simulink model "B2_SIM"  (R2024a)
settings: Solver=VariableStepAuto  StartTime=0.0  StopTime=1200  RelTol=1e-3
values from neighbouring files (symbols this model uses):
  alpha1 = 0.03198    [diseased_prm.m]
  alpha2 = 0.05591    [diseased_prm.m]
  beta1 = 0.008275    [diseased_prm.m]
  beta2 = 0.03255    [diseased_prm.m]
  CaCO2_IC = 0.565    [diseased_prm.m]
  CaO2_IC = 0.184    [diseased_prm.m]
  CsatCO2 = 1.9488    [diseased_prm.m]
  CsatO2 = 0.2128    [diseased_prm.m]
  CvCO2_IC = 0.602    [diseased_prm.m]
  CvO2_IC = 0.134    [diseased_prm.m]
  h1 = 0.3836    [diseased_prm.m]
  h2 = 1.819    [diseased_prm.m]
  K = 11.5620    (= 11.562)    [B2.m]
  K1 = 15.0    (= 15)    [diseased_prm.m]
  K2 = 194.4    [diseased_prm.m]
  kEff = 0.55    [diseased_prm.m]
  kem = 0.192    [diseased_prm.m]
  MRCO2 = 3.30/1000    (= 0.0033)    [diseased_prm.m]
  MRO2 = 3.80/1000    (= 0.0038)    [diseased_prm.m]
  PACO2_IC = 55.0    (= 55)    [diseased_prm.m]
  PAO2_IC = 57.0    (= 57)    [diseased_prm.m]
  Patm = 760.0    (= 760)    [diseased_prm.m]
  PdCO2_IC = 53.0    (= 53)    [diseased_prm.m]
  PdO2_IC = 60.0    (= 60)    [diseased_prm.m]
  PECO2_IC = 40.0    (= 40)    [diseased_prm.m]
  PEO2_IC = 200.0    (= 200)    [diseased_prm.m]
  PICO2 = (Patm - Pws)*FICO2    (= 0)    [diseased_prm.m]
  PIO2 = (Patm - Pws)*FIO2    (= 713)    [diseased_prm.m]
  Pws = 47.0    (= 47)    [diseased_prm.m]
  R = 10.0    (= 10)    [diseased_prm.m]
  Rlung = 1.4013    [diseased_prm.m]
  Rtube = 3.76    [diseased_prm.m]
  shunt = 36.5/100    (= 0.365)    [diseased_prm.m]
  Tau_LT = 18.0    (= 18)    [diseased_prm.m]
  Tau_TL = 10.0    (= 10)    [diseased_prm.m]
  Tsamp = 1e-3    (= 0.001)    [diseased_prm.m]
  VD = 0.15    [diseased_prm.m]
  VECO2 = 1.5    [diseased_prm.m]
  VEO2 = 1.5    [diseased_prm.m]
  VprimeEcmo = 0.08    [B2.m]
  VReference = 0.2    [B2.m]    (also in diseased_prm.m = 0.6)
  VTCO2 = 6000/1000    (= 6)    [diseased_prm.m]
  VTO2 = 7700/1000    (= 7.7)    [diseased_prm.m]
libraries: fl_lib x14, nesl_utility x7, slpidlib x4, ee_lib x2
settings Model: Creator=seman  LastModifiedBy=seman

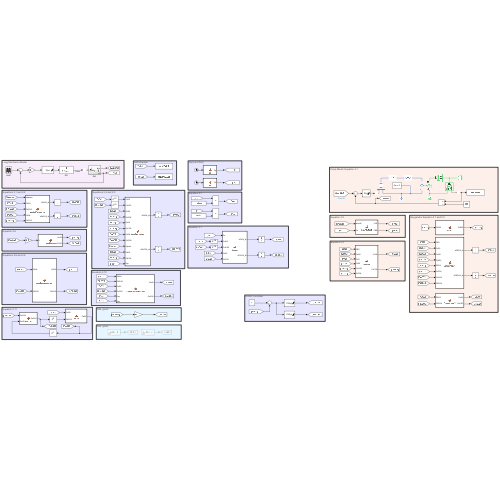
[thumbnail: Simulink's stored preview of the top-level diagram]
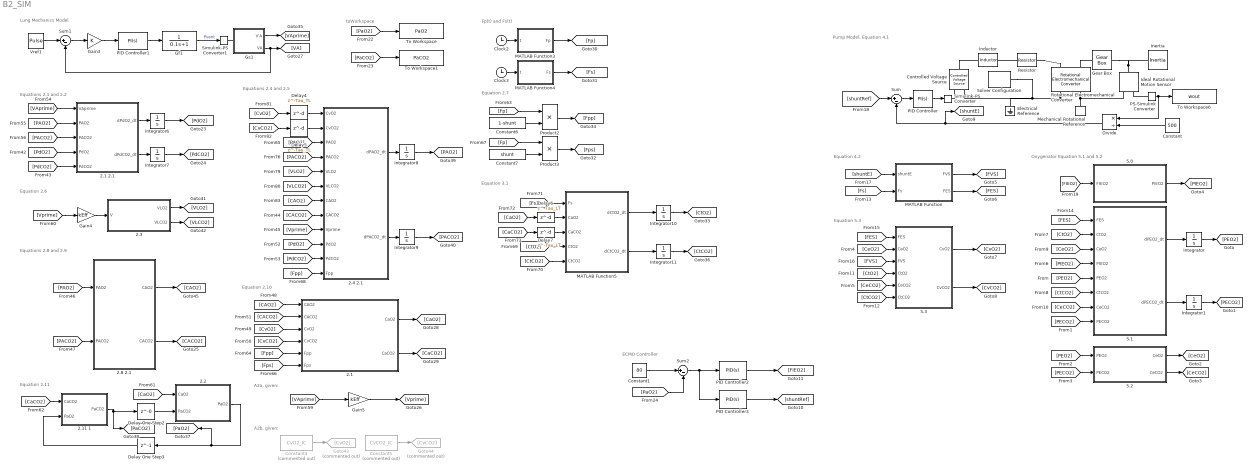
== system B2_SIM ==
  note: ECMO Controller
  note: Equation 5.3
  note: Oxygenator Equation 5.1 and 5.2
  note: Equation 4.2
  note: Equation 2.7
  note: Lung Mechanics Model
  note: Equation 2.6
  note: Equations 2.8 and 2.9
  note: A2b, given:
  note: Equation 2.11
  note: toWorkspace
  note: Fp(t) and Fs(t)
  note: Equations 2.1 and 2.2
  note: Equations 2.4 and 2.5
  note: Equation 3.1
  note: Equation 2.10
  note: A2a, given:
  note: Pump Model, Equation 4.1
  " 2.11 1" : MATLAB Function  TreatAsAtomicUnit=on  SystemSampleTime=Tsamp
  2.1 : MATLAB Function  TreatAsAtomicUnit=on  SystemSampleTime=Tsamp
  2.1 2.1 : MATLAB Function  TreatAsAtomicUnit=on  SystemSampleTime=Tsamp
  2.2 : MATLAB Function  TreatAsAtomicUnit=on  SystemSampleTime=Tsamp
  2.3 : MATLAB Function  TreatAsAtomicUnit=on  SystemSampleTime=Tsamp
  2.4 2.1 : MATLAB Function  TreatAsAtomicUnit=on  SystemSampleTime=Tsamp
  2.8 2.1 : MATLAB Function  TreatAsAtomicUnit=on  SystemSampleTime=Tsamp
  5.0 : MATLAB Function  TreatAsAtomicUnit=on  SystemSampleTime=Tsamp
  5.1 : MATLAB Function  TreatAsAtomicUnit=on  SystemSampleTime=Tsamp
  5.2 : MATLAB Function  TreatAsAtomicUnit=on  SystemSampleTime=Tsamp
  5.3 : MATLAB Function  TreatAsAtomicUnit=on  SystemSampleTime=Tsamp
  Clock2 : Clock
  Clock3 : Clock
  Constant : Constant  Value=500
  Constant1 : Constant  Value=80
  Constant4 : Constant  Commented=on  Value=CvO2_IC  SampleTime=Tsamp
  Constant5 : Constant  Commented=on  Value=CvCO2_IC  SampleTime=Tsamp
  Constant6 : Constant  Value=1-shunt
  Constant7 : Constant  Value=shunt
  Controlled Voltage Source : fl_lib/Electrical/Electrical Sources/Controlled Voltage Source
  Delay One Step2 : Delay  DelayLength=0  InitialCondition=PACO2_IC  SampleTime=Tsamp
  Delay One Step3 : Delay  DelayLength=1  InitialCondition=PAO2_IC  SampleTime=Tsamp
  Delay4 : Delay  DelayLength=Tau_TL  InitialCondition=CvO2_IC  SampleTime=Tsamp
  Delay5 : Delay  DelayLength=Tau_TL  InitialCondition=CvCO2_IC  SampleTime=Tsamp
  Delay6 : Delay  DelayLength=Tau_LT  InitialCondition=CaO2_IC  SampleTime=Tsamp
  Delay7 : Delay  DelayLength=Tau_LT  InitialCondition=CaCO2_IC  SampleTime=Tsamp
  Divide : Product  Inputs=*/
  Electrical Reference : fl_lib/Electrical/Electrical Elements/Electrical Reference
  Gain3 : Gain  Gain=K
  Gain4 : Gain  Gain=kEff
  Gain5 : Gain  Gain=kEff
  Gear Box : fl_lib/Mechanical/Mechanisms/Gear Box  ratio=Ng  t_in_specify=off  t_in_priority=None  t_in=0 N*m  t_in_nominal_specify=off  t_in_nominal_value=1  t_in_nominal_unit=N*m  t_out_specify=off  t_out_priority=None  t_out=0 N*m  t_out_nominal_specify=off  t_out_nominal_value=1  t_out_nominal_unit=N*m
  Gf1 : TransferFcn  Denominator=[0.1 1]
  Goto43 : Goto  Commented=on  GotoTag=CvO2
  Goto44 : Goto  Commented=on  GotoTag=CvCO2
  Gs1 : Subsystem
      settings: PortSchema="{\"entries\":[{\"content\":{\"sides\":[{\"content\":{\"connectorIds\":[\"Out1\",\"Out2\"]},\"type\":\"ConnectorPlacement.EquallySpacedRectSide\",\"uuid\":\"c27d9928-4b86-4da3-a78c-9004074cc1dc\"},{\"content\":{\"connectorIds\":[\"RConn1\"],\"side\":\"RIGHT\"},\"type\":\"ConnectorPlacement.EquallySpacedRectSide\",\"uuid\":\"e53dfbe0-a76d-428f-9787-aeb453f7ae86\"},{\"content\":{\"side\":\"TOP\"},\"type\":\"ConnectorPlacement.EquallySpacedRectSide\",\"uuid\":\"62f67270-c149-475e-8334-fb9ed6626660\"}]},\"type\":\"ConnectorPlacement.EquallySpacedConnector\",\"uuid\":\"79b18274-f0e6-497d-aef4-92df5a9879dd\"}],\"packageUris\":[\"http://schema.mathworks.com/mf0/Connector/R2020b\"],\"version\":\"1.0\"}"
  Ideal Rotational Motion Sensor : fl_lib/Mechanical/Mechanical Sensors/Ideal Rotational Motion Sensor  reference=foundation.enum.MeasurementReference.difference  acceleration_port=false  velocity_port=true  position_port=false  wrap_angle=false  offset=0 rad
      settings: InternalSimscapePortConfiguration="{\"Bottom\":[],\"Left\":[{\"id\":\"R\",\"label\":\"R\",\"type\":\"foundation.mechanical.rotational.rotational\"}],\"Right\":[{\"id\":\"C\",\"label\":\"C\",\"type\":\"foundation.mechanical.rotational.rotational\"},{\"id\":\"W\",\"label\":\"W\",\"type\":\"output\"}],\"Top\":[]}"
  Inductor : ee_lib/Passive/Inductor  l=L mH  enable_L_tol=ee.enum.toleranceApplication.none  L_tol=20  tol_distribution=ee.enum.toleranceDistribution.uniform  nSigma=4  r=0 Ohm  g=1e-9 1/Ohm  enable_operating_limits=ee.enum.enable.no  operating_limit_action=ee.enum.passive.reportOpLim.warn  max_working_current=1 A  power_rating=1 W  enable_faults=ee.enum.enable.no  fault_action=simscape.enum.assert.action.none  lambdaPercent=50  k_faulted=0.9999  turnsShort=ee.enum.passive.inductor.turnsShortOption.no  openCct=ee.enum.enable.no  groundShort=ee.enum.passive.inductor.groundShortOption.no  groundShortG=0 1/Ohm  tau_fault=1e-3 s  fault_trigger=ee.enum.faults.faultTrigger.temporal  t_fault=1 s  max_permissible_voltage=100 V  n_fail_on_voltage=1  max_permissible_current=1 A  t_fail_on_current=1 s  i_L_specify=off  i_L_priority=High  i_L=0 A  i_L_nominal_specify=off  i_L_nominal_value=1  i_L_nominal_unit=A  faulted_specify=off  faulted_priority=None  faulted=0
  Inertia : fl_lib/Mechanical/Rotational Elements/Inertia  inertia=JL kg*m^2  num_ports=foundation.enum.numPorts2.one  w_specify=off  w_priority=High  w=0 rad/s  w_nominal_specify=off  w_nominal_value=1  w_nominal_unit=rad/s  t_specify=off  t_priority=None  t=0 N*m  t_nominal_specify=off  t_nominal_value=1  t_nominal_unit=N*m
  Integrator : Integrator  InitialCondition=PEO2_IC
  Integrator1 : Integrator  InitialCondition=PECO2_IC
  Integrator10 : Integrator  InitialCondition=CvO2_IC
  Integrator11 : Integrator  InitialCondition=CvCO2_IC
  Integrator6 : Integrator  InitialCondition=PdO2_IC
  Integrator7 : Integrator  InitialCondition=PdCO2_IC
  Integrator8 : Integrator  InitialCondition=PAO2_IC
  Integrator9 : Integrator  InitialCondition=PACO2_IC
  MATLAB Function : MATLAB Function  TreatAsAtomicUnit=on  SystemSampleTime=Tsamp
  MATLAB Function3 : MATLAB Function  TreatAsAtomicUnit=on  SystemSampleTime=Tsamp
  MATLAB Function4 : MATLAB Function  TreatAsAtomicUnit=on  SystemSampleTime=Tsamp
  MATLAB Function5 : MATLAB Function  TreatAsAtomicUnit=on  SystemSampleTime=Tsamp
  Mechanical Rotational Reference : fl_lib/Mechanical/Rotational Elements/Mechanical Rotational Reference
  PID Controller : slpidlib/PID Controller  Controller=PI  Form=Parallel  TimeDomain=Continuous-time  UseExternalTs=off  SampleTime=-1  IntegratorMethod=Forward Euler  FilterMethod=Forward Euler  ControllerParametersSource=internal  P=24.7  I=48.35  UseKiTs=off  D=0  UseExternalDerivativeSource=off  N=100  UseFilter=on  TunerSelectOption=Transfer Function Based (PID Tuner App)  InitialConditionSource=internal  InitialConditionForIntegrator=0  InitialConditionForFilter=0  DifferentiatorICPrevScaledInput=0  ExternalReset=none  TrackingMode=off  Kt=1  LimitOutput=on  SatLimitsSource=internal  UpperSaturationLimit=48  LowerSaturationLimit=0  LinearizeAsGain=on  AntiWindupMode=none  Kb=1  LimitIntegrator=off  UpperIntegratorSaturationLimit=inf  LowerIntegratorSaturationLimit=-inf  POutMin=[]  POutMax=[]  IOutMin=[]  IOutMax=[]  DOutMin=[]  DOutMax=[]  NOutMin=[]  NOutMax=[]  SumOutMin=[]  SumOutMax=[]  SaturationOutMin=[]  SaturationOutMax=[]  PParamMin=[]  PParamMax=[]  IParamMin=[]  IParamMax=[]  DParamMin=[]  DParamMax=[]  NParamMin=[]  NParamMax=[]  KbParamMin=[]  KbParamMax=[]  KtParamMin=[]  KtParamMax=[]  KbOutMin=[]  KbOutMax=[]  KtOutMin=[]  KtOutMax=[]  IntegratorOutMin=[]  IntegratorOutMax=[]  FilterOutMin=[]  FilterOutMax=[]  SumI1OutMin=[]  SumI1OutMax=[]  SumI2OutMin=[]  SumI2OutMax=[]  SumI3OutMin=[]  SumI3OutMax=[]  SumI4OutMin=[]  SumI4OutMax=[]  SumDOutMin=[]  SumDOutMax=[]  DifferentiatorOutMin=[]  DifferentiatorOutMax=[]  FilterDiffOutCoefMin=[]  FilterDiffOutCoefMax=[]  ReciprocalOutMin=[]  ReciprocalOutMax=[]  SumDenOutMin=[]  SumDenOutMax=[]  SumNumOutMin=[]  SumNumOutMax=[]  DivideOutMin=[]  DivideOutMax=[]  UdiffTsProdOutMin=[]  UdiffTsProdOutMax=[]  NTsProdOutMin=[]  NTsProdOutMax=[]  UintegralTsProdOutMin=[]  UintegralTsProdOutMax=[]  UngainTsProdOutMin=[]  UngainTsProdOutMax=[]  ClampingZeroOutDataTypeStr=Inherit: Inherit via back propagation  ClampingZeroOutMin=[]  ClampingZeroOutMax=[]  FilterDenConstantOutDataTypeStr=Inherit: Inherit via back propagation  FilterDenConstantOutMin=[]  FilterDenConstantOutMax=[]  PCopyOutDataTypeStr=Inherit: Inherit via back propagation  PCopyOutMin=[]  PCopyOutMax=[]  NCopyOutDataTypeStr=Inherit: Inherit via back propagation  NCopyOutMin=[]  NCopyOutMax=[]  IntegratorContinuousStateAttributes=''  IntegratorStateMustResolveToSignalObject=off  IntegratorRTWStateStorageClass=Auto  FilterContinuousStateAttributes=''  FilterStateMustResolveToSignalObject=off  FilterRTWStateStorageClass=Auto  ParallelPVariant=InternalParameters  IdealPVariant=Disabled  IVariant=InternalParameters  DVariant=Disabled  IntegratorVariant=Continuous  SatVariant=Enabled  AWVariant=Passthrough  PCopyVariant=Disabled  TRVariant=Disabled  FdbkBlocksVariant=Forward  IdealPFdbkVariant=Disabled  SatFdbkVariant=Disabled  DerivativeFilterVariant=Disabled  NVariant=Disabled  NCopyVariant=Disabled_SignalSpec  FilterICVariant=Disabled  IntegratorICVariant=InternalICs  ExternalResetVariant=Disabled  TRSumVariant=Passthrough  SumFdbkVariant=Disabled  SumVariant=Sum_PI  TsampFilterVariant=InternalTs  TsampNgainVariant=Passthrough  TsampIntegralVariant=Disabled_SignalSpec  ExternalSaturationOutDataTypeStr=Inherit: Same as second input  DerivativeSourceVariant=Disabled
  PID Controller1 : slpidlib/PID Controller  Controller=PI  Form=Parallel  TimeDomain=Continuous-time  UseExternalTs=off  SampleTime=-1  IntegratorMethod=Forward Euler  FilterMethod=Forward Euler  ControllerParametersSource=internal  P=1  I=3.125  UseKiTs=off  D=0  UseExternalDerivativeSource=off  N=100  UseFilter=on  TunerSelectOption=Transfer Function Based (PID Tuner App)  InitialConditionSource=internal  InitialConditionForIntegrator=0  InitialConditionForFilter=0  DifferentiatorICPrevScaledInput=0  ExternalReset=none  TrackingMode=off  Kt=1  LimitOutput=on  SatLimitsSource=internal  UpperSaturationLimit=inf  LowerSaturationLimit=0  LinearizeAsGain=on  AntiWindupMode=back-calculation  Kb=1  LimitIntegrator=off  UpperIntegratorSaturationLimit=inf  LowerIntegratorSaturationLimit=-inf  POutMin=[]  POutMax=[]  IOutMin=[]  IOutMax=[]  DOutMin=[]  DOutMax=[]  NOutMin=[]  NOutMax=[]  SumOutMin=[]  SumOutMax=[]  SaturationOutMin=[]  SaturationOutMax=[]  PParamMin=[]  PParamMax=[]  IParamMin=[]  IParamMax=[]  DParamMin=[]  DParamMax=[]  NParamMin=[]  NParamMax=[]  KbParamMin=[]  KbParamMax=[]  KtParamMin=[]  KtParamMax=[]  KbOutMin=[]  KbOutMax=[]  KtOutMin=[]  KtOutMax=[]  IntegratorOutMin=[]  IntegratorOutMax=[]  FilterOutMin=[]  FilterOutMax=[]  SumI1OutMin=[]  SumI1OutMax=[]  SumI2OutMin=[]  SumI2OutMax=[]  SumI3OutMin=[]  SumI3OutMax=[]  SumI4OutMin=[]  SumI4OutMax=[]  SumDOutMin=[]  SumDOutMax=[]  DifferentiatorOutMin=[]  DifferentiatorOutMax=[]  FilterDiffOutCoefMin=[]  FilterDiffOutCoefMax=[]  ReciprocalOutMin=[]  ReciprocalOutMax=[]  SumDenOutMin=[]  SumDenOutMax=[]  SumNumOutMin=[]  SumNumOutMax=[]  DivideOutMin=[]  DivideOutMax=[]  UdiffTsProdOutMin=[]  UdiffTsProdOutMax=[]  NTsProdOutMin=[]  NTsProdOutMax=[]  UintegralTsProdOutMin=[]  UintegralTsProdOutMax=[]  UngainTsProdOutMin=[]  UngainTsProdOutMax=[]  ClampingZeroOutDataTypeStr=Inherit: Inherit via back propagation  ClampingZeroOutMin=[]  ClampingZeroOutMax=[]  FilterDenConstantOutDataTypeStr=Inherit: Inherit via back propagation  FilterDenConstantOutMin=[]  FilterDenConstantOutMax=[]  PCopyOutDataTypeStr=Inherit: Inherit via back propagation  PCopyOutMin=[]  PCopyOutMax=[]  NCopyOutDataTypeStr=Inherit: Inherit via back propagation  NCopyOutMin=[]  NCopyOutMax=[]  IntegratorContinuousStateAttributes=''  IntegratorStateMustResolveToSignalObject=off  IntegratorRTWStateStorageClass=Auto  FilterContinuousStateAttributes=''  FilterStateMustResolveToSignalObject=off  FilterRTWStateStorageClass=Auto  ParallelPVariant=InternalParameters  IdealPVariant=Disabled  IVariant=InternalParameters  DVariant=Disabled  IntegratorVariant=Continuous  SatVariant=Enabled  AWVariant=BackCalculation  PCopyVariant=Disabled  TRVariant=Disabled  FdbkBlocksVariant=Forward  IdealPFdbkVariant=Disabled  SatFdbkVariant=Disabled  DerivativeFilterVariant=Disabled  NVariant=Disabled  NCopyVariant=Disabled_SignalSpec  FilterICVariant=Disabled  IntegratorICVariant=InternalICs  ExternalResetVariant=Disabled  TRSumVariant=Passthrough  SumFdbkVariant=Disabled  SumVariant=Sum_PI  TsampFilterVariant=InternalTs  TsampNgainVariant=Passthrough  TsampIntegralVariant=Disabled_SignalSpec  ExternalSaturationOutDataTypeStr=Inherit: Same as second input  DerivativeSourceVariant=Disabled
  PID Controller2 : slpidlib/PID Controller  Controller=PID  Form=Parallel  TimeDomain=Continuous-time  UseExternalTs=off  SampleTime=-1  IntegratorMethod=Forward Euler  FilterMethod=Forward Euler  ControllerParametersSource=internal  P=1  I=0.1  UseKiTs=off  D=0.2  UseExternalDerivativeSource=off  N=100  UseFilter=on  TunerSelectOption=Transfer Function Based (PID Tuner App)  InitialConditionSource=internal  InitialConditionForIntegrator=0.2  InitialConditionForFilter=0.2  DifferentiatorICPrevScaledInput=0  ExternalReset=none  TrackingMode=off  Kt=1  LimitOutput=on  SatLimitsSource=internal  UpperSaturationLimit=1  LowerSaturationLimit=0.2  LinearizeAsGain=on  AntiWindupMode=none  Kb=1  LimitIntegrator=off  UpperIntegratorSaturationLimit=inf  LowerIntegratorSaturationLimit=-inf  POutMin=[]  POutMax=[]  IOutMin=[]  IOutMax=[]  DOutMin=[]  DOutMax=[]  NOutMin=[]  NOutMax=[]  SumOutMin=[]  SumOutMax=[]  SaturationOutMin=[]  SaturationOutMax=[]  PParamMin=[]  PParamMax=[]  IParamMin=[]  IParamMax=[]  DParamMin=[]  DParamMax=[]  NParamMin=[]  NParamMax=[]  KbParamMin=[]  KbParamMax=[]  KtParamMin=[]  KtParamMax=[]  KbOutMin=[]  KbOutMax=[]  KtOutMin=[]  KtOutMax=[]  IntegratorOutMin=[]  IntegratorOutMax=[]  FilterOutMin=[]  FilterOutMax=[]  SumI1OutMin=[]  SumI1OutMax=[]  SumI2OutMin=[]  SumI2OutMax=[]  SumI3OutMin=[]  SumI3OutMax=[]  SumI4OutMin=[]  SumI4OutMax=[]  SumDOutMin=[]  SumDOutMax=[]  DifferentiatorOutMin=[]  DifferentiatorOutMax=[]  FilterDiffOutCoefMin=[]  FilterDiffOutCoefMax=[]  ReciprocalOutMin=[]  ReciprocalOutMax=[]  SumDenOutMin=[]  SumDenOutMax=[]  SumNumOutMin=[]  SumNumOutMax=[]  DivideOutMin=[]  DivideOutMax=[]  UdiffTsProdOutMin=[]  UdiffTsProdOutMax=[]  NTsProdOutMin=[]  NTsProdOutMax=[]  UintegralTsProdOutMin=[]  UintegralTsProdOutMax=[]  UngainTsProdOutMin=[]  UngainTsProdOutMax=[]  ClampingZeroOutDataTypeStr=Inherit: Inherit via back propagation  ClampingZeroOutMin=[]  ClampingZeroOutMax=[]  FilterDenConstantOutDataTypeStr=Inherit: Inherit via back propagation  FilterDenConstantOutMin=[]  FilterDenConstantOutMax=[]  PCopyOutDataTypeStr=Inherit: Inherit via back propagation  PCopyOutMin=[]  PCopyOutMax=[]  NCopyOutDataTypeStr=Inherit: Inherit via back propagation  NCopyOutMin=[]  NCopyOutMax=[]  IntegratorContinuousStateAttributes=''  IntegratorStateMustResolveToSignalObject=off  IntegratorRTWStateStorageClass=Auto  FilterContinuousStateAttributes=''  FilterStateMustResolveToSignalObject=off  FilterRTWStateStorageClass=Auto  ParallelPVariant=InternalParameters  IdealPVariant=Disabled  IVariant=InternalParameters  DVariant=InternalParameters  IntegratorVariant=Continuous  SatVariant=Enabled  AWVariant=Passthrough  PCopyVariant=Disabled  TRVariant=Disabled  FdbkBlocksVariant=Forward  IdealPFdbkVariant=Disabled  SatFdbkVariant=Disabled  DerivativeFilterVariant=ContFilter  NVariant=InternalParameters  NCopyVariant=Disabled  FilterICVariant=InternalICsFilter  IntegratorICVariant=InternalICs  ExternalResetVariant=Disabled  TRSumVariant=Passthrough  SumFdbkVariant=Disabled  SumVariant=Sum_PID  TsampFilterVariant=InternalTs  TsampNgainVariant=Passthrough  TsampIntegralVariant=Disabled_SignalSpec  ExternalSaturationOutDataTypeStr=Inherit: Same as second input  DerivativeSourceVariant=ErrorSignal
  PID Controller3 : slpidlib/PID Controller  Controller=PID  Form=Parallel  TimeDomain=Continuous-time  UseExternalTs=off  SampleTime=-1  IntegratorMethod=Forward Euler  FilterMethod=Forward Euler  ControllerParametersSource=internal  P=10  I=0.1  UseKiTs=off  D=0.2  UseExternalDerivativeSource=off  N=100  UseFilter=on  TunerSelectOption=Transfer Function Based (PID Tuner App)  InitialConditionSource=internal  InitialConditionForIntegrator=0.2  InitialConditionForFilter=0.2  DifferentiatorICPrevScaledInput=0  ExternalReset=none  TrackingMode=off  Kt=1  LimitOutput=on  SatLimitsSource=internal  UpperSaturationLimit=1  LowerSaturationLimit=0.2  LinearizeAsGain=on  AntiWindupMode=none  Kb=1  LimitIntegrator=off  UpperIntegratorSaturationLimit=inf  LowerIntegratorSaturationLimit=-inf  POutMin=[]  POutMax=[]  IOutMin=[]  IOutMax=[]  DOutMin=[]  DOutMax=[]  NOutMin=[]  NOutMax=[]  SumOutMin=[]  SumOutMax=[]  SaturationOutMin=[]  SaturationOutMax=[]  PParamMin=[]  PParamMax=[]  IParamMin=[]  IParamMax=[]  DParamMin=[]  DParamMax=[]  NParamMin=[]  NParamMax=[]  KbParamMin=[]  KbParamMax=[]  KtParamMin=[]  KtParamMax=[]  KbOutMin=[]  KbOutMax=[]  KtOutMin=[]  KtOutMax=[]  IntegratorOutMin=[]  IntegratorOutMax=[]  FilterOutMin=[]  FilterOutMax=[]  SumI1OutMin=[]  SumI1OutMax=[]  SumI2OutMin=[]  SumI2OutMax=[]  SumI3OutMin=[]  SumI3OutMax=[]  SumI4OutMin=[]  SumI4OutMax=[]  SumDOutMin=[]  SumDOutMax=[]  DifferentiatorOutMin=[]  DifferentiatorOutMax=[]  FilterDiffOutCoefMin=[]  FilterDiffOutCoefMax=[]  ReciprocalOutMin=[]  ReciprocalOutMax=[]  SumDenOutMin=[]  SumDenOutMax=[]  SumNumOutMin=[]  SumNumOutMax=[]  DivideOutMin=[]  DivideOutMax=[]  UdiffTsProdOutMin=[]  UdiffTsProdOutMax=[]  NTsProdOutMin=[]  NTsProdOutMax=[]  UintegralTsProdOutMin=[]  UintegralTsProdOutMax=[]  UngainTsProdOutMin=[]  UngainTsProdOutMax=[]  ClampingZeroOutDataTypeStr=Inherit: Inherit via back propagation  ClampingZeroOutMin=[]  ClampingZeroOutMax=[]  FilterDenConstantOutDataTypeStr=Inherit: Inherit via back propagation  FilterDenConstantOutMin=[]  FilterDenConstantOutMax=[]  PCopyOutDataTypeStr=Inherit: Inherit via back propagation  PCopyOutMin=[]  PCopyOutMax=[]  NCopyOutDataTypeStr=Inherit: Inherit via back propagation  NCopyOutMin=[]  NCopyOutMax=[]  IntegratorContinuousStateAttributes=''  IntegratorStateMustResolveToSignalObject=off  IntegratorRTWStateStorageClass=Auto  FilterContinuousStateAttributes=''  FilterStateMustResolveToSignalObject=off  FilterRTWStateStorageClass=Auto  ParallelPVariant=InternalParameters  IdealPVariant=Disabled  IVariant=InternalParameters  DVariant=InternalParameters  IntegratorVariant=Continuous  SatVariant=Enabled  AWVariant=Passthrough  PCopyVariant=Disabled  TRVariant=Disabled  FdbkBlocksVariant=Forward  IdealPFdbkVariant=Disabled  SatFdbkVariant=Disabled  DerivativeFilterVariant=ContFilter  NVariant=InternalParameters  NCopyVariant=Disabled  FilterICVariant=InternalICsFilter  IntegratorICVariant=InternalICs  ExternalResetVariant=Disabled  TRSumVariant=Passthrough  SumFdbkVariant=Disabled  SumVariant=Sum_PID  TsampFilterVariant=InternalTs  TsampNgainVariant=Passthrough  TsampIntegralVariant=Disabled_SignalSpec  ExternalSaturationOutDataTypeStr=Inherit: Same as second input  DerivativeSourceVariant=ErrorSignal
  PS-Simulink Converter : nesl_utility/PS-Simulink Converter  PhysicalDomain=network_engine_domain  SubClassName=ps_output  LeftPortType=input  RightPortType=output  PseudoPeriodic=off  Frequencies=[]  VectorFormat=inherit  Unit=inherit  AffineConversion=off
  Product2 : Product
  Product3 : Product
  Resistor : ee_lib/Passive/Resistor  R=R Ohm  enable_R_tol=ee.enum.toleranceApplication.none  R_tol=5  tol_distribution=ee.enum.toleranceDistribution.uniform  nSigma=4  enable_operating_limits=ee.enum.enable.no  operating_limit_action=ee.enum.passive.reportOpLim.warn  power_rating=1 W  max_working_voltage=100 V  enable_faults=ee.enum.enable.no  fault_action=simscape.enum.assert.action.none  R_faulted=inf Ohm  fault_trigger=ee.enum.faults.faultTrigger.temporal  t_fault=1 s  max_permissible_current=1 A  t_fail_on_current=1 s  noise_mode=ee.enum.sources.noise.Disabled  Tdevice=25 degC  sample_time=1e-3 s  repeatability=ee.enum.ic.repeatability.notRepeatable  user_seed=0  auto_seed=3922919431  faulted_specify=off  faulted_priority=None  faulted=0  power_derating_T1=70 degC  power_derating_T2=155 degC  operating_temperature_range_vec=[-50, 150] degC  alpha=3.93e-3 1/K  Tmeas=25 degC  thermal_mass=100 J/K  temperature_specify=off  temperature_priority=High  temperature=298.15 K  temperature_nominal_specify=off  temperature_nominal_value=1  temperature_nominal_unit=K
  Rotational Electromechanical Converter : fl_lib/Electrical/Electrical Elements/Rotational Electromechanical Converter  K=kem V*s/rad  i_specify=off  i_priority=None  i=0 A  i_nominal_specify=off  i_nominal_value=1  i_nominal_unit=A  v_specify=off  v_priority=None  v=0 V  v_nominal_specify=off  v_nominal_value=1  v_nominal_unit=V  t_specify=off  t_priority=None  t=0 N*m  t_nominal_specify=off  t_nominal_value=1  t_nominal_unit=N*m  w_specify=off  w_priority=None  w=0 rad/s  w_nominal_specify=off  w_nominal_value=1  w_nominal_unit=rad/s
  Simulink-PS Converter : nesl_utility/Simulink-PS Converter  PhysicalDomain=network_engine_domain  SubClassName=ps_input  LeftPortType=input  RightPortType=output  PseudoPeriodic=off  Frequencies=[]  NoiseDistribution=none  NoiseParameters=[]  Unit=1  AffineConversion=off  FilteringAndDerivatives=provide  SimscapeFilterOrder=1  InputFilterTimeConstant=0.001  UdotUserProvided=0
  Simulink-PS Converter1 : nesl_utility/Simulink-PS Converter  PhysicalDomain=network_engine_domain  SubClassName=ps_input  LeftPortType=input  RightPortType=output  PseudoPeriodic=off  Frequencies=[]  NoiseDistribution=none  NoiseParameters=[]  Unit=1  AffineConversion=off  FilteringAndDerivatives=provide  SimscapeFilterOrder=1  InputFilterTimeConstant=0.001  UdotUserProvided=0
  Solver Configuration : nesl_utility/Solver Configuration  PhysicalDomain=network_engine_domain  SubClassName=solver  LeftPortType=input  RightPortType=generic  Tones=[]  Harmonics=[]  SimulateNoise=off  Profile=off  UseLocalSampling=off  EnableSwitchedLinearOptims=on  FrequencyDomain=off  UseCCode=off  RelTol=0.001  AbsTol=0.001  MinStep=1e-09  ToWorkspace=off  RevertToSquareIcSolve=off  NumHomotopyIterations=100  PhasorMode=off  PhasorModeNumHarmonics=1  ConsistencySolver=NEWTON_XTOL_AFTER_FTOL  IndexReductionMethod=DerivativeReplacement  DoDC=off  ResidualTolerance=1e-09  ConsistencyTolSource=GLOBAL  ConsistencyAbsTol=0.001  ConsistencyRelTol=0.001  ConsistencyTolFactor=0.001  UseLocalSolver=off  LocalSolverChoice=NE_BACKWARD_EULER_ADVANCER  ResolveIndetEquations=on  FunctionEvalNumThread=1  LocalSolverSampleTime=0.001  DoFixedCost=off  MaxNonlinIter=3  MaxModeIter=2  ComputeImpulses=off  ImpulseIterations=2  LinearAlgebra=auto  LinearAlgebraNumThread=0  EquationFormulation=NE_TIME_EF  DelaysMemoryBudget=1024  AutomaticFiltering=on  FilteringTimeConstant=0.001  PartitionStorageMethod=AS_NEEDED  PartitionMemoryBudget=1024  PartitionMethod=ROBUST  MultibodyUseLocalSolver=off  MultibodyLocalSolverChoice=ODE1  MultibodyLocalSolverSampleTime=0.001
  Sum : Sum  Inputs=|+-
  Sum1 : Sum  Inputs=|+-
  Sum2 : Sum  Inputs=|+-
  To Workspace : ToWorkspace  VariableName=PaO2  SaveFormat=Timeseries  SampleTime=Tsamp
  To Workspace1 : ToWorkspace  VariableName=PaCO2  SaveFormat=Timeseries  SampleTime=Tsamp
  To Workspace6 : ToWorkspace  VariableName=wout  SaveFormat=Timeseries  SampleTime=Tsamp
  Vref1 : DiscretePulseGenerator  PulseType=Time based  Amplitude=VReference  Period=1/0.2  PulseWidth=35
  wires:
  [PACO2] -> 2.4 2.1/4(PACO2)
  [CtO2] -> MATLAB Function5/4(CtO2)
  Sum1/1 -> Gain3/1
  [CaO2] -> 2.2/1(CaO2)
  MATLAB Function4/1(Fs) -> [Fs]
  " 2.11 1"/1(PaCO2) -> Delay One Step2/1, [PaCO2]
  [VLCO2] -> 2.4 2.1/6(VLCO2)
  Integrator6/1 -> [PdO2]
  [PaCO2] -> To Workspace1/1
  Constant6/1 -> Product2/2
  Delay7/1 -> MATLAB Function5/3(CaCO2)
  Gain5/1 -> [Vprime]
  [Vprime] -> 2.4 2.1/9(Vprime)
  2.4 2.1/1(dPAO2_dt) -> Integrator8/1
  Integrator8/1 -> [PAO2]
  [PaO2] -> To Workspace/1
  [PdCO2] -> 2.4 2.1/11(PdCO2)
  [Fp] -> Product3/1
  Integrator11/1 -> [CtCO2]
  [CAO2] -> 2.4 2.1/7(CAO2)
  2.2/1(PaO2) -> Delay One Step3/1, [PaO2]
  Product3/1 -> [Fps]
  [PAO2] -> 2.4 2.1/3(PAO2)
  2.4 2.1/2(dPACO2_dt) -> Integrator9/1
  [CvCO2] -> 2.1/4(CvCO2)
  2.3/1(VLO2) -> [VLO2]
  Constant7/1 -> Product3/2
  [VAprime] -> Gain5/1
  [PACO2] -> 2.1 2.1/3(PACO2)
  Product2/1 -> [Fpp]
  [CvO2] -> 2.1/3(CvO2)
  Constant5/1 -> Goto44/1
  2.1 2.1/2(dPdCO2_dt) -> Integrator7/1
  [VLO2] -> 2.4 2.1/5(VLO2)
  Gs1/2(VA) -> Sum1/2, [VA]
  [Vprime] -> Gain4/1
  Delay One Step3/1 -> " 2.11 1"/2(PaO2)
  Vref1/1 -> Sum1/1
  Gain3/1 -> PID Controller1/1
  [VAprime] -> 2.1 2.1/1(VAprime)
  Constant4/1 -> Goto43/1
  MATLAB Function5/1(dCtO2_dt) -> Integrator10/1
  Clock2/1 -> MATLAB Function3/1(t)
  2.3/2(VLCO2) -> [VLCO2]
  Integrator9/1 -> [PACO2]
  [CAO2] -> 2.1/1(CAO2)
  [CaCO2] -> Delay7/1
  Gain4/1 -> 2.3/1(V)
  [PAO2] -> 2.1 2.1/2(PAO2)
  Delay One Step2/1 -> 2.2/2(PaCO2)
  Gs1/1(V'A) -> [VAprime]
  [CvCO2] -> Delay5/1
  Delay6/1 -> MATLAB Function5/2(CaO2)
  [CACO2] -> 2.1/2(CACO2)
  Integrator7/1 -> [PdCO2]
  2.8 2.1/1(CAO2) -> [CAO2]
  [CaCO2] -> " 2.11 1"/1(CaCO2)
  2.8 2.1/2(CACO2) -> [CACO2]
  MATLAB Function3/1(Fp) -> [Fp]
  Gf1/1 -> Simulink-PS Converter1/1  "Pvent"
  2.1/2(CaCO2) -> [CaCO2]
  [CaO2] -> Delay6/1
  [CtCO2] -> MATLAB Function5/5(CtCO2)
  2.1/1(CaO2) -> [CaO2]
  [PAO2] -> 2.8 2.1/1(PAO2)
  Integrator10/1 -> [CtO2]
  [PACO2] -> 2.8 2.1/2(PACO2)
  [Fp] -> Product2/1
  Clock3/1 -> MATLAB Function4/1(t)
  [CvO2] -> Delay4/1
  [Fpp] -> 2.1/5(Fpp)
  [PdO2] -> 2.4 2.1/10(PdO2)
  MATLAB Function5/2(dCtCO2_dt) -> Integrator11/1
  2.1 2.1/1(dPdO2_dt) -> Integrator6/1
  [Fpp] -> 2.4 2.1/12(Fpp)
  [PdCO2] -> 2.1 2.1/5(PdCO2)
  Delay5/1 -> 2.4 2.1/2(CvCO2)
  [Fps] -> 2.1/6(Fps)
  [CACO2] -> 2.4 2.1/8(CACO2)
  [PdO2] -> 2.1 2.1/4(PdO2)
  [Fs] -> MATLAB Function5/1(Fs)
  PID Controller1/1 -> Gf1/1
  Delay4/1 -> 2.4 2.1/1(CvO2)
  5.1/1(dPEO2_dt) -> Integrator/1
  5.1/2(dPECO2_dt) -> Integrator1/1
  Integrator/1 -> [PEO2]
  Integrator1/1 -> [PECO2]
  [PEO2] -> 5.1/5(PEO2)
  [PECO2] -> 5.1/8(PECO2)
  [PEO2] -> 5.2/1(PEO2)
  [PECO2] -> 5.2/2(PECO2)
  5.2/1(CeO2) -> [CeO2]
  5.2/2(CeCO2) -> [CeCO2]
  [CeO2] -> 5.3/2(CeO2)
  [CeCO2] -> 5.3/5(CeCO2)
  [PIEO2] -> 5.1/4(PIEO2)
  [CtO2] -> 5.1/2(CtO2)
  [CtCO2] -> 5.1/6(CtCO2)
  [CeO2] -> 5.1/3(CeO2)
  [CeCO2] -> 5.1/7(CeCO2)
  [CtO2] -> 5.3/4(CtO2)
  [CtCO2] -> 5.3/6(CtCO2)
  [Fs] -> MATLAB Function/2(Fs)
  MATLAB Function/1(FVS) -> [FVS]
  MATLAB Function/2(FES) -> [FES]
  [FES] -> 5.1/1(FES)
  [FES] -> 5.3/1(FES)
  [FVS] -> 5.3/3(FVS)
  5.3/1(CvO2) -> [CvO2]
  5.3/2(CvCO2) -> [CvCO2]
  [shuntE] -> MATLAB Function/1(shuntE)
  Constant/1 -> Divide/2
  PS-Simulink Converter/1 -> Divide/1, To Workspace6/1
  PID Controller/1 -> Simulink-PS Converter/1
  Sum/1 -> PID Controller/1
  Divide/1 -> [shuntE], Sum/2
  5.0/1(PIEO2) -> [PIEO2]
  [shuntRef] -> Sum/1
  [FIEO2] -> 5.0/1(FIEO2)
  Constant1/1 -> Sum2/1
  Sum2/1 -> PID Controller3/1, PID Controller2/1
  [PaO2] -> Sum2/2
  PID Controller2/1 -> [FIEO2]
  PID Controller3/1 -> [shuntRef]
  connections:
  Gs1/RConn1 -- Simulink-PS Converter1/RConn1
  Ideal Rotational Motion Sensor/LConn1 -- Gear Box/RConn1 -- Inertia/LConn1
  Rotational Electromechanical Converter/RConn1 -- Solver Configuration/RConn1 -- Controlled Voltage Source/RConn2 -- Electrical Reference/LConn1
  Rotational Electromechanical Converter/RConn2 -- Mechanical Rotational Reference/LConn1 -- Ideal Rotational Motion Sensor/RConn1
  Controlled Voltage Source/LConn1 -- Inductor/LConn1
  Rotational Electromechanical Converter/LConn2 -- Gear Box/LConn1
  PS-Simulink Converter/LConn1 -- Ideal Rotational Motion Sensor/RConn2
  Resistor/RConn1 -- Rotational Electromechanical Converter/LConn1
  Controlled Voltage Source/RConn1 -- Simulink-PS Converter/RConn1
  Resistor/LConn1 -- Inductor/RConn1

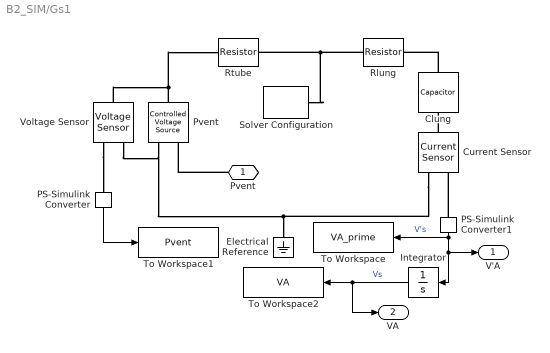
== system B2_SIM/Gs1 ==
  Clung : fl_lib/Electrical/Electrical Elements/Capacitor  c=Clung F  r=0 Ohm  g=0 1/Ohm  i_specify=off  i_priority=None  i=0 A  i_nominal_specify=off  i_nominal_value=1  i_nominal_unit=A  v_specify=off  v_priority=None  v=0 V  v_nominal_specify=off  v_nominal_value=1  v_nominal_unit=V  vc_specify=off  vc_priority=High  vc=0 V  vc_nominal_specify=off  vc_nominal_value=1  vc_nominal_unit=V
  Current Sensor : fl_lib/Electrical/Electrical Sensors/Current Sensor
  Electrical Reference : fl_lib/Electrical/Electrical Elements/Electrical Reference
  Integrator : Integrator
  PS-Simulink Converter : nesl_utility/PS-Simulink Converter  PhysicalDomain=network_engine_domain  SubClassName=ps_output  LeftPortType=input  RightPortType=output  PseudoPeriodic=off  Frequencies=[]  VectorFormat=inherit  Unit=inherit  AffineConversion=off
  PS-Simulink Converter1 : nesl_utility/PS-Simulink Converter  PhysicalDomain=network_engine_domain  SubClassName=ps_output  LeftPortType=input  RightPortType=output  PseudoPeriodic=off  Frequencies=[]  VectorFormat=inherit  Unit=inherit  AffineConversion=off
  Pvent : fl_lib/Electrical/Electrical Sources/Controlled Voltage Source
  Rlung : fl_lib/Electrical/Electrical Elements/Resistor  R=Rlung Ohm  i_specify=off  i_priority=None  i=0 A  i_nominal_specify=off  i_nominal_value=1  i_nominal_unit=A  v_specify=off  v_priority=None  v=0 V  v_nominal_specify=off  v_nominal_value=1  v_nominal_unit=V
  Rtube : fl_lib/Electrical/Electrical Elements/Resistor  R=Rtube Ohm  i_specify=off  i_priority=None  i=0 A  i_nominal_specify=off  i_nominal_value=1  i_nominal_unit=A  v_specify=off  v_priority=None  v=0 V  v_nominal_specify=off  v_nominal_value=1  v_nominal_unit=V
  Solver Configuration : nesl_utility/Solver Configuration  PhysicalDomain=network_engine_domain  SubClassName=solver  LeftPortType=input  RightPortType=generic  Tones=[]  Harmonics=[]  SimulateNoise=off  Profile=off  UseLocalSampling=off  EnableSwitchedLinearOptims=on  FrequencyDomain=off  UseCCode=off  RelTol=0.001  AbsTol=0.001  MinStep=1e-09  ToWorkspace=off  RevertToSquareIcSolve=off  NumHomotopyIterations=100  PhasorMode=off  PhasorModeNumHarmonics=1  ConsistencySolver=NEWTON_XTOL_AFTER_FTOL  IndexReductionMethod=DerivativeReplacement  DoDC=off  ResidualTolerance=1e-09  ConsistencyTolSource=GLOBAL  ConsistencyAbsTol=0.001  ConsistencyRelTol=0.001  ConsistencyTolFactor=0.001  UseLocalSolver=off  LocalSolverChoice=NE_BACKWARD_EULER_ADVANCER  ResolveIndetEquations=on  FunctionEvalNumThread=1  LocalSolverSampleTime=0.001  DoFixedCost=off  MaxNonlinIter=3  MaxModeIter=2  ComputeImpulses=off  ImpulseIterations=2  LinearAlgebra=auto  LinearAlgebraNumThread=0  EquationFormulation=NE_TIME_EF  DelaysMemoryBudget=1024  AutomaticFiltering=on  FilteringTimeConstant=0.001  PartitionStorageMethod=AS_NEEDED  PartitionMemoryBudget=1024  PartitionMethod=ROBUST  MultibodyUseLocalSolver=off  MultibodyLocalSolverChoice=ODE1  MultibodyLocalSolverSampleTime=0.001
  To Workspace : ToWorkspace  VariableName=VA_prime  SaveFormat=Timeseries  SampleTime=-1
  To Workspace1 : ToWorkspace  VariableName=Pvent  SaveFormat=Timeseries  SampleTime=-1
  To Workspace2 : ToWorkspace  VariableName=VA  SaveFormat=Timeseries  SampleTime=-1
  Voltage Sensor : fl_lib/Electrical/Electrical Sensors/Voltage Sensor
  " Pvent " : PMIOPort  Side=Right
  V'A : Outport
  VA : Outport  Port=2
  wires:
  PS-Simulink Converter/1 -> To Workspace1/1
  Integrator/1 -> VA/1, To Workspace2/1  "Vs"
  PS-Simulink Converter1/1 -> V'A/1, Integrator/1, To Workspace/1  "V's"
  connections:
  Current Sensor/RConn2 -- Pvent/RConn2 -- Voltage Sensor/RConn2 -- Electrical Reference/LConn1
  Voltage Sensor/RConn1 -- PS-Simulink Converter/LConn1
  Current Sensor/LConn1 -- Clung/RConn1
  Rlung/LConn1 -- Solver Configuration/RConn1 -- Rtube/RConn1
  Clung/LConn1 -- Rlung/RConn1
  Pvent/LConn1 -- Voltage Sensor/LConn1 -- Rtube/LConn1
  PS-Simulink Converter1/LConn1 -- Current Sensor/RConn1
  " Pvent "/RConn1 -- Pvent/RConn1

== matlab function B2_SIM/ 2.11 1 ==
  data: CaCO2 input; PaO2 input; PaCO2 output; K2 parameter; beta2 parameter; alpha2 parameter; h2 parameter; CsatCO2 parameter
function PaCO2  = PaCO2(CaCO2, PaO2, K2, beta2, alpha2, h2, CsatCO2)
    PaCO2 = K2 * (1 + alpha2*PaO2)  / (1 + beta2*PaO2)  * ( CaCO2/(CsatCO2 - CaCO2))^h2;
end

== matlab function B2_SIM/2.2 ==
  data: PaO2 output; CaO2 input; alpha1 parameter; beta1 parameter; K1 parameter; PaCO2 input; h1 parameter; CsatO2 parameter
function PaO2 = PaO2(CaO2, alpha1, beta1, K1, PaCO2, h1, CsatO2)
    PaO2 =  K1 * (1 + alpha1*PaCO2) / (1 + beta1*PaCO2) * ( CaO2 /(CsatO2 -  CaO2 ))^h1;
end

== matlab function B2_SIM/MATLAB Function4 ==
  data: t input; Fs output
function Fs = fcn(t)
    u = mod(t, 0.84);  % Sawtooth wave (0 to period)
    if (0 < u) && (u < 0.19)
        Fs = (1 + 670*(sin(pi*u/0.19))^2) / 1000;
    else
        Fs = 1/1000;
    end
end

== matlab function B2_SIM/MATLAB Function5 ==
  data: dCtO2_dt output; Fs input; CaO2 input; CaCO2 input; CtO2 input; CtCO2 input; dCtCO2_dt output; MRO2 parameter; MRCO2 parameter; VTO2 parameter; VTCO2 parameter
function [dCtO2_dt, dCtCO2_dt] = tissue(Fs, CaO2, CaCO2, CtO2, CtCO2, MRO2, MRCO2, VTO2, VTCO2)
    dCtO2_dt = (-MRO2 + Fs * (CaO2 - CtO2)) / VTO2;
    dCtCO2_dt = (MRCO2 + Fs * (CaCO2 - CtCO2)) /VTCO2;
end

== matlab function B2_SIM/5.1 ==
  data: dPEO2_dt output; FES input; CtO2 input; CeO2 input; PIEO2 input; PEO2 input; CtCO2 input; CeCO2 input; PECO2 input; dPECO2_dt output; VprimeEcmo parameter; VEO2 parameter; VECO2 parameter
function [dPEO2_dt, dPECO2_dt] = Oxygenator1(FES, CtO2, CeO2, PIEO2, PEO2, CtCO2, CeCO2, PECO2, VprimeEcmo, VEO2, VECO2)
    dPEO2_dt = (863*FES*(CtO2 - CeO2) + VprimeEcmo*(PIEO2 - PEO2))/VEO2;
    dPECO2_dt = (863*FES*(CtCO2 - CeCO2) - VprimeEcmo*PECO2)/VECO2;
end

== matlab function B2_SIM/5.0 ==
  data: PIEO2 output; Pws parameter; FIEO2 input; Patm parameter
function PIEO2 = pieo2(Pws, FIEO2, Patm)
    PIEO2 = (Patm - Pws)*FIEO2;
end

== matlab function B2_SIM/5.2 ==
  data: CeO2 output; PEO2 input; PECO2 input; CeCO2 output; beta1 parameter; beta2 parameter; K1 parameter; K2 parameter; h1 parameter; h2 parameter; alpha1 parameter; alpha2 parameter; CsatO2 parameter; CsatCO2 parameter
function [CeO2, CeCO2] = Oxygenator2(PEO2, PECO2, beta1, beta2, K1, K2, h1, h2, alpha1, alpha2, CsatO2, CsatCO2)
    CeO2 = CsatO2 * (PEO2/K1*(1+beta1*PECO2)/(1+alpha1*PECO2))^(1/h1) / (1 + (PEO2/K1*(1+beta1*PECO2)/(1+alpha1*PECO2))^(1/h1)); 
    CeCO2 = CsatCO2 * (PECO2/K2*(1+beta2*PEO2)/(1+alpha2*PEO2))^(1/h2) / (1 + (PECO2/K2*(1+beta2*PEO2)/(1+alpha2*PEO2))^(1/h2)); 
end

== matlab function B2_SIM/5.3 ==
  data: FES input; CvO2 output; CeO2 input; FVS input; CtO2 input; CeCO2 input; CtCO2 input; CvCO2 output
function [CvO2, CvCO2] = venous(FES, CeO2, FVS, CtO2, CeCO2, CtCO2)
    CvO2 = (FES*CeO2 + FVS*CtO2) / (FES + FVS);
    CvCO2 = (FES*CeCO2 + FVS*CtCO2) / (FES + FVS);
end

== matlab function B2_SIM/MATLAB Function ==
  data: shuntE input; FVS output; Fs input; FES output
function [FVS, FES] = shuntEffect(shuntE, Fs)
    FVS = (1-shuntE)*Fs;
    FES = shuntE*Fs;
end

== matlab function B2_SIM/2.4 2.1 ==
  data: CvO2 input; CvCO2 input; PAO2 input; PACO2 input; dPAO2_dt output; dPACO2_dt output; VLO2 input; VLCO2 input; CAO2 input; CACO2 input; Vprime input; PdO2 input; PdCO2 input; Fpp input
function [dPAO2_dt, dPACO2_dt] = gasExchange(CvO2, CvCO2, PAO2, PACO2, VLO2, VLCO2, CAO2, CACO2, Vprime, PdO2, PdCO2, Fpp)
    if Vprime > 0
        dPAO2_dt  = ( 863*Fpp*(CvO2-CAO2)   + Vprime*(PdO2-PAO2))    /VLO2;
        dPACO2_dt = ( 863*Fpp*(CvCO2-CACO2) + Vprime*(PdCO2-PACO2))  /VLCO2;
    else
        dPAO2_dt  = (863*Fpp*(CvO2-CAO2))   /VLO2;
        dPACO2_dt = (863*Fpp*(CvCO2-CACO2)) /VLCO2;
    end
end

== matlab function B2_SIM/2.1 2.1 ==
  data: VAprime input; dPdO2_dt output; PAO2 input; PACO2 input; PdO2 input; PdCO2 input; dPdCO2_dt output; PIO2 parameter; PICO2 parameter; VD parameter
function [dPdO2_dt, dPdCO2_dt] = partialPressures(VAprime, PAO2, PACO2, PdO2, PdCO2, PIO2, PICO2, VD)
    if VAprime > 0
        dPdO2_dt = VAprime * (PIO2 - PdO2) / VD;
        dPdCO2_dt = VAprime * (PICO2 - PdCO2) / VD;
    else
        dPdO2_dt = VAprime * (PdO2 - PAO2) / VD;
        dPdCO2_dt = VAprime * (PdCO2 - PACO2) / VD;
    end
end

== matlab function B2_SIM/2.3 ==
  data: V input; VLO2 output; VLCO2 output; VL0 parameter
function [VLO2, VLCO2] = lungStorage(V, VL0)
    VLO2 = VL0 + V;
    VLCO2 = 1.28 * VLO2;
end

== matlab function B2_SIM/2.1 ==
  data: CaO2 output; CAO2 input; CACO2 input; CvO2 input; CvCO2 input; CaCO2 output; Fpp input; Fps input
function [CaO2, CaCO2] = arterialConcentrations(CAO2, CACO2, CvO2, CvCO2, Fpp, Fps)
   CaO2 = (Fpp*CAO2 + Fps*CvO2)/(Fpp + Fps);
   CaCO2 = (Fpp*CACO2 + Fps*CvCO2)/(Fpp + Fps);
end

== matlab function B2_SIM/2.8 2.1 ==
  data: K2 parameter; beta1 parameter; CAO2 output; CACO2 output; beta2 parameter; K1 parameter; alpha1 parameter; alpha2 parameter; CsatO2 parameter; CsatCO2 parameter; h1 parameter; h2 parameter; PAO2 input; PACO2 input
function [CAO2, CACO2] = gasConsentration(K2, beta1, beta2, K1, alpha1, alpha2, CsatO2, CsatCO2, h1, h2, PAO2, PACO2)
    CAO2 = CsatO2 * ( ( PAO2 / K1 * ( 1 + beta1*PACO2 )/( 1 + alpha1*PACO2 ) ) ^(1/h1) ...
               / (1 + ( PAO2 / K1 * ( 1 + beta1*PACO2 )/( 1 + alpha1*PACO2 ) ) ^(1/h1)));
    
    CACO2 = CsatCO2 * ( ( PACO2 / K2 * ( 1 + beta2*PAO2 )/( 1 + alpha2*PAO2 ) ) ^(1/h2) ...
               / (1 +   ( PACO2 / K2 * ( 1 + beta2*PAO2 )/( 1 + alpha2*PAO2 ) ) ^(1/h2)));
end

== matlab function B2_SIM/MATLAB Function3 ==
  data: t input; Fp output
function Fp = fcn(t)
    u = mod(t, 0.84);
    if (0 < u) && (u < 0.25)
        Fp = (1+ 460*(sin(pi*u/0.25))^1.55) / 1000;
    else
        Fp = 1 / 1000;
    end
end
